simulink model "P702_NI_SoftECU"  (R2019a)
settings: Solver=ode1  StartTime=0.0  StopTime=Inf  FixedStep=0.001  RelTol=1e-3  EnableMultiTasking=on
PreLoadFcn:
  | run '.\VeriStand_BlockSet\NIVeriStandAddPaths.m'
undefined symbols (not defined in the file or in its folder): magnitude
libraries: simulink x83, simulink_extras x1
(part 6 of 76)

== system P702_NI_SoftECU/Input/ABS_ESC/DesiredTorqBrk_2_0x214 ==
  Bus_Sig : BusCreator  Inputs=7
  PrplWhlRear_Tq_RqMn : S-Function  Priority=1  FunctionName=NIVeriStandIO  Parameters=width dtype portnum stime stype btype  SFunctionDeploymentMode=off  EnableBusSupport=off  mask(NI VeriStand Inport){portnum=1, width=-1, stime=-1, dtype=auto, stype=auto, btype=1}
      mask prompts: portnum "Port number:"; width "Port dimensions (-1 for dynamically sized):"; stime "Sample time (-1 for inherited):"; dtype "Data type:"; stype "Signal type:"; btype "Block type:"
      mask help: Use this inport on any level of nested subsystems to allow NI VeriStand software to map signals to it.
      mask init:
      | NIVeriStandIO_init;
      settings: CopyFcn=NIVeriStand_MDL_functions('', 'IO_copy');  DeleteFcn=NIVeriStand_MDL_functions('', 'IO_delete');  MoveFcn=set_param(gcb, 'Mask', 'on');
      mask Callback portnum: NIVeriStand_MDL_functions('', 'IO_setportnum');
      mask TypeOptions dtype: auto | double | single | int8 | uint8 | int16 | uint16 | int32 | uint32 | boolean
      mask Callback dtype: NIVeriStand_MDL_functions('', 'IO_booleansignal');
      mask TypeOptions stype: auto | real | complex
      mask Display:
      | patch([-x x], [-y y], [.90980 .81960 .32156]);
      | plot([xrad -x x xrad], [yrad -y y yrad]);
      | fprintf('NI In%d', portnum);
  PrplWhlRear_Tq_RqMx : S-Function  Priority=2  FunctionName=NIVeriStandIO  Parameters=width dtype portnum stime stype btype  SFunctionDeploymentMode=off  EnableBusSupport=off  mask(NI VeriStand Inport){portnum=2, width=-1, stime=-1, dtype=auto, stype=auto, btype=1}
      mask prompts: portnum "Port number:"; width "Port dimensions (-1 for dynamically sized):"; stime "Sample time (-1 for inherited):"; dtype "Data type:"; stype "Signal type:"; btype "Block type:"
      mask help: Use this inport on any level of nested subsystems to allow NI VeriStand software to map signals to it.
      mask init:
      | NIVeriStandIO_init;
      settings: CopyFcn=NIVeriStand_MDL_functions('', 'IO_copy');  DeleteFcn=NIVeriStand_MDL_functions('', 'IO_delete');  MoveFcn=set_param(gcb, 'Mask', 'on');
      mask Callback portnum: NIVeriStand_MDL_functions('', 'IO_setportnum');
      mask TypeOptions dtype: auto | double | single | int8 | uint8 | int16 | uint16 | int32 | uint32 | boolean
      mask Callback dtype: NIVeriStand_MDL_functions('', 'IO_booleansignal');
      mask TypeOptions stype: auto | real | complex
      mask Display:
      | patch([-x x], [-y y], [.90980 .81960 .32156]);
      | plot([xrad -x x xrad], [yrad -y y yrad]);
      | fprintf('NI In%d', portnum);
  PrplWhlTot_Tq_RqMn : S-Function  Priority=3  FunctionName=NIVeriStandIO  Parameters=width dtype portnum stime stype btype  SFunctionDeploymentMode=off  EnableBusSupport=off  mask(NI VeriStand Inport){portnum=3, width=-1, stime=-1, dtype=auto, stype=auto, btype=1}
      mask prompts: portnum "Port number:"; width "Port dimensions (-1 for dynamically sized):"; stime "Sample time (-1 for inherited):"; dtype "Data type:"; stype "Signal type:"; btype "Block type:"
      mask help: Use this inport on any level of nested subsystems to allow NI VeriStand software to map signals to it.
      mask init:
      | NIVeriStandIO_init;
      settings: CopyFcn=NIVeriStand_MDL_functions('', 'IO_copy');  DeleteFcn=NIVeriStand_MDL_functions('', 'IO_delete');  MoveFcn=set_param(gcb, 'Mask', 'on');
      mask Callback portnum: NIVeriStand_MDL_functions('', 'IO_setportnum');
      mask TypeOptions dtype: auto | double | single | int8 | uint8 | int16 | uint16 | int32 | uint32 | boolean
      mask Callback dtype: NIVeriStand_MDL_functions('', 'IO_booleansignal');
      mask TypeOptions stype: auto | real | complex
      mask Display:
      | patch([-x x], [-y y], [.90980 .81960 .32156]);
      | plot([xrad -x x xrad], [yrad -y y yrad]);
      | fprintf('NI In%d', portnum);
  PrplWhlTqRqMn_No_Cnt : S-Function  Priority=4  FunctionName=NIVeriStandIO  Parameters=width dtype portnum stime stype btype  SFunctionDeploymentMode=off  EnableBusSupport=off  mask(NI VeriStand Inport){portnum=4, width=-1, stime=-1, dtype=auto, stype=auto, btype=1}
      mask prompts: portnum "Port number:"; width "Port dimensions (-1 for dynamically sized):"; stime "Sample time (-1 for inherited):"; dtype "Data type:"; stype "Signal type:"; btype "Block type:"
      mask help: Use this inport on any level of nested subsystems to allow NI VeriStand software to map signals to it.
      mask init:
      | NIVeriStandIO_init;
      settings: CopyFcn=NIVeriStand_MDL_functions('', 'IO_copy');  DeleteFcn=NIVeriStand_MDL_functions('', 'IO_delete');  MoveFcn=set_param(gcb, 'Mask', 'on');
      mask Callback portnum: NIVeriStand_MDL_functions('', 'IO_setportnum');
      mask TypeOptions dtype: auto | double | single | int8 | uint8 | int16 | uint16 | int32 | uint32 | boolean
      mask Callback dtype: NIVeriStand_MDL_functions('', 'IO_booleansignal');
      mask TypeOptions stype: auto | real | complex
      mask Display:
      | patch([-x x], [-y y], [.90980 .81960 .32156]);
      | plot([xrad -x x xrad], [yrad -y y yrad]);
      | fprintf('NI In%d', portnum);
  PrplWhlTqRqMn_No_Cs : S-Function  Priority=5  FunctionName=NIVeriStandIO  Parameters=width dtype portnum stime stype btype  SFunctionDeploymentMode=off  EnableBusSupport=off  mask(NI VeriStand Inport){portnum=5, width=-1, stime=-1, dtype=auto, stype=auto, btype=1}
      mask prompts: portnum "Port number:"; width "Port dimensions (-1 for dynamically sized):"; stime "Sample time (-1 for inherited):"; dtype "Data type:"; stype "Signal type:"; btype "Block type:"
      mask help: Use this inport on any level of nested subsystems to allow NI VeriStand software to map signals to it.
      mask init:
      | NIVeriStandIO_init;
      settings: CopyFcn=NIVeriStand_MDL_functions('', 'IO_copy');  DeleteFcn=NIVeriStand_MDL_functions('', 'IO_delete');  MoveFcn=set_param(gcb, 'Mask', 'on');
      mask Callback portnum: NIVeriStand_MDL_functions('', 'IO_setportnum');
      mask TypeOptions dtype: auto | double | single | int8 | uint8 | int16 | uint16 | int32 | uint32 | boolean
      mask Callback dtype: NIVeriStand_MDL_functions('', 'IO_booleansignal');
      mask TypeOptions stype: auto | real | complex
      mask Display:
      | patch([-x x], [-y y], [.90980 .81960 .32156]);
      | plot([xrad -x x xrad], [yrad -y y yrad]);
      | fprintf('NI In%d', portnum);
  RgenBrkDynoMde_B_Actl : S-Function  Priority=6  FunctionName=NIVeriStandIO  Parameters=width dtype portnum stime stype btype  SFunctionDeploymentMode=off  EnableBusSupport=off  mask(NI VeriStand Inport){portnum=6, width=-1, stime=-1, dtype=auto, stype=auto, btype=1}
      mask prompts: portnum "Port number:"; width "Port dimensions (-1 for dynamically sized):"; stime "Sample time (-1 for inherited):"; dtype "Data type:"; stype "Signal type:"; btype "Block type:"
      mask help: Use this inport on any level of nested subsystems to allow NI VeriStand software to map signals to it.
      mask init:
      | NIVeriStandIO_init;
      settings: CopyFcn=NIVeriStand_MDL_functions('', 'IO_copy');  DeleteFcn=NIVeriStand_MDL_functions('', 'IO_delete');  MoveFcn=set_param(gcb, 'Mask', 'on');
      mask Callback portnum: NIVeriStand_MDL_functions('', 'IO_setportnum');
      mask TypeOptions dtype: auto | double | single | int8 | uint8 | int16 | uint16 | int32 | uint32 | boolean
      mask Callback dtype: NIVeriStand_MDL_functions('', 'IO_booleansignal');
      mask TypeOptions stype: auto | real | complex
      mask Display:
      | patch([-x x], [-y y], [.90980 .81960 .32156]);
      | plot([xrad -x x xrad], [yrad -y y yrad]);
      | fprintf('NI In%d', portnum);
  RgenTqFalt_B_Actl : S-Function  Priority=7  FunctionName=NIVeriStandIO  Parameters=width dtype portnum stime stype btype  SFunctionDeploymentMode=off  EnableBusSupport=off  mask(NI VeriStand Inport){portnum=7, width=-1, stime=-1, dtype=auto, stype=auto, btype=1}
      mask prompts: portnum "Port number:"; width "Port dimensions (-1 for dynamically sized):"; stime "Sample time (-1 for inherited):"; dtype "Data type:"; stype "Signal type:"; btype "Block type:"
      mask help: Use this inport on any level of nested subsystems to allow NI VeriStand software to map signals to it.
      mask init:
      | NIVeriStandIO_init;
      settings: CopyFcn=NIVeriStand_MDL_functions('', 'IO_copy');  DeleteFcn=NIVeriStand_MDL_functions('', 'IO_delete');  MoveFcn=set_param(gcb, 'Mask', 'on');
      mask Callback portnum: NIVeriStand_MDL_functions('', 'IO_setportnum');
      mask TypeOptions dtype: auto | double | single | int8 | uint8 | int16 | uint16 | int32 | uint32 | boolean
      mask Callback dtype: NIVeriStand_MDL_functions('', 'IO_booleansignal');
      mask TypeOptions stype: auto | real | complex
      mask Display:
      | patch([-x x], [-y y], [.90980 .81960 .32156]);
      | plot([xrad -x x xrad], [yrad -y y yrad]);
      | fprintf('NI In%d', portnum);
  DesiredTorqBrk_2_0x214 : Outport
  wires:
  RgenBrkDynoMde_B_Actl/1 -> Bus_Sig/7  "RgenBrkDynoMde_B_Actl"
  RgenTqFalt_B_Actl/1 -> Bus_Sig/6  "RgenTqFalt_B_Actl"
  PrplWhlTqRqMn_No_Cnt/1 -> Bus_Sig/5  "PrplWhlTqRqMn_No_Cnt"
  PrplWhlTqRqMn_No_Cs/1 -> Bus_Sig/4  "PrplWhlTqRqMn_No_Cs"
  PrplWhlRear_Tq_RqMn/1 -> Bus_Sig/3  "PrplWhlRear_Tq_RqMn"
  PrplWhlRear_Tq_RqMx/1 -> Bus_Sig/2  "PrplWhlRear_Tq_RqMx"
  PrplWhlTot_Tq_RqMn/1 -> Bus_Sig/1  "PrplWhlTot_Tq_RqMn"
  Bus_Sig/1 -> DesiredTorqBrk_2_0x214/1  "DesiredTorqBrk_2_0x214"

== system P702_NI_SoftECU/Input/ABS_ESC/Global_PATS_SubTarget_0x49 ==
  Bus_Sig : BusCreator  Inputs=2
  immoSubTarget1Cmd_T1 : Constant  Commented=on  Value=0
  immoSubTarget1Data_T1 : Constant  Commented=on  Value=0
  Global_PATS_SubTarget_0x49 : Outport
  wires:
  immoSubTarget1Data_T1/1 -> Bus_Sig/2  "immoSubTarget1Data_T1"
  immoSubTarget1Cmd_T1/1 -> Bus_Sig/1  "immoSubTarget1Cmd_T1"
  Bus_Sig/1 -> Global_PATS_SubTarget_0x49/1  "Global_PATS_SubTarget_0x49"

== system P702_NI_SoftECU/Input/ABS_ESC/SelectDriveModeData2_0x44E ==
  Bus_Sig : BusCreator  Inputs=12
  SelDrvMdePos01_D_Stat : Constant  Commented=on  Value=31
  SelDrvMdePos02_D_Stat : Constant  Commented=on  Value=31
  SelDrvMdePos03_D_Stat : Constant  Commented=on  Value=31
  SelDrvMdePos04_D_Stat : Constant  Commented=on  Value=31
  SelDrvMdePos05_D_Stat : Constant  Commented=on  Value=31
  SelDrvMdePos06_D_Stat : Constant  Commented=on  Value=31
  SelDrvMdePos07_D_Stat : Constant  Commented=on  Value=31
  SelDrvMdePos08_D_Stat : Constant  Commented=on  Value=31
  SelDrvMdePos09_D_Stat : Constant  Commented=on  Value=31
  SelDrvMdePos10_D_Stat : Constant  Commented=on  Value=31
  SelDrvMdePos11_D_Stat : Constant  Commented=on  Value=31
  SelDrvMdePos12_D_Stat : Constant  Commented=on  Value=31
  SelectDriveModeData2_0x44E : Outport
  wires:
  SelDrvMdePos08_D_Stat/1 -> Bus_Sig/12  "SelDrvMdePos08_D_Stat"
  SelDrvMdePos09_D_Stat/1 -> Bus_Sig/11  "SelDrvMdePos09_D_Stat"
  SelDrvMdePos10_D_Stat/1 -> Bus_Sig/10  "SelDrvMdePos10_D_Stat"
  SelDrvMdePos11_D_Stat/1 -> Bus_Sig/9  "SelDrvMdePos11_D_Stat"
  SelDrvMdePos12_D_Stat/1 -> Bus_Sig/8  "SelDrvMdePos12_D_Stat"
  SelDrvMdePos07_D_Stat/1 -> Bus_Sig/7  "SelDrvMdePos07_D_Stat"
  SelDrvMdePos06_D_Stat/1 -> Bus_Sig/6  "SelDrvMdePos06_D_Stat"
  SelDrvMdePos05_D_Stat/1 -> Bus_Sig/5  "SelDrvMdePos05_D_Stat"
  SelDrvMdePos04_D_Stat/1 -> Bus_Sig/4  "SelDrvMdePos04_D_Stat"
  SelDrvMdePos03_D_Stat/1 -> Bus_Sig/3  "SelDrvMdePos03_D_Stat"
  SelDrvMdePos02_D_Stat/1 -> Bus_Sig/2  "SelDrvMdePos02_D_Stat"
  SelDrvMdePos01_D_Stat/1 -> Bus_Sig/1  "SelDrvMdePos01_D_Stat"
  Bus_Sig/1 -> SelectDriveModeData2_0x44E/1  "SelectDriveModeData2_0x44E"

== system P702_NI_SoftECU/Input/ABS_ESC/SelectDriveModeData_0x420 ==
  ActvDrvMde_D2_Stat : Constant  Commented=on  Value=31
  AwdMde_D_RqBrk : Constant  Commented=on  Value=5
  Bus_Sig : BusCreator  Inputs=18
  SelDrvMdeMsgTxt_D_Rq : Constant  Commented=on  Value=0
  SelDrvMdePos01_B_Avail : Constant  Commented=on  Value=0
  SelDrvMdePos02_B_Avail : Constant  Commented=on  Value=0
  SelDrvMdePos03_B_Avail : Constant  Commented=on  Value=0
  SelDrvMdePos04_B_Avail : Constant  Commented=on  Value=0
  SelDrvMdePos05_B_Avail : Constant  Commented=on  Value=0
  SelDrvMdePos06_B_Avail : Constant  Commented=on  Value=0
  SelDrvMdePos07_B_Avail : Constant  Commented=on  Value=0
  SelDrvMdePos08_B_Avail : Constant  Commented=on  Value=0
  SelDrvMdePos09_B_Avail : Constant  Commented=on  Value=0
  SelDrvMdePos10_B_Avail : Constant  Commented=on  Value=0
  SelDrvMdePos11_B_Avail : Constant  Commented=on  Value=0
  SelDrvMdePos12_B_Avail : Constant  Commented=on  Value=0
  SelDrvMdePt_D_Rq : Constant  Commented=on  Value=0
  SelDrvMde_D2_Rq : Constant  Commented=on  Value=31
  SelDrvMde_D_Stat : Constant  Commented=on  Value=0
  SelectDriveModeData_0x420 : Outport
  wires:
  SelDrvMde_D2_Rq/1 -> Bus_Sig/18  "SelDrvMde_D2_Rq"
  ActvDrvMde_D2_Stat/1 -> Bus_Sig/17  "ActvDrvMde_D2_Stat"
  SelDrvMdePos12_B_Avail/1 -> Bus_Sig/16  "SelDrvMdePos12_B_Avail"
  SelDrvMdePos11_B_Avail/1 -> Bus_Sig/15  "SelDrvMdePos11_B_Avail"
  SelDrvMdePos10_B_Avail/1 -> Bus_Sig/14  "SelDrvMdePos10_B_Avail"
  SelDrvMdePos09_B_Avail/1 -> Bus_Sig/13  "SelDrvMdePos09_B_Avail"
  SelDrvMdePos08_B_Avail/1 -> Bus_Sig/12  "SelDrvMdePos08_B_Avail"
  SelDrvMdePos07_B_Avail/1 -> Bus_Sig/11  "SelDrvMdePos07_B_Avail"
  SelDrvMdePos06_B_Avail/1 -> Bus_Sig/10  "SelDrvMdePos06_B_Avail"
  SelDrvMdePos05_B_Avail/1 -> Bus_Sig/9  "SelDrvMdePos05_B_Avail"
  SelDrvMdePos04_B_Avail/1 -> Bus_Sig/8  "SelDrvMdePos04_B_Avail"
  SelDrvMdePos03_B_Avail/1 -> Bus_Sig/7  "SelDrvMdePos03_B_Avail"
  SelDrvMdePos02_B_Avail/1 -> Bus_Sig/6  "SelDrvMdePos02_B_Avail"
  AwdMde_D_RqBrk/1 -> Bus_Sig/5  "AwdMde_D_RqBrk"
  SelDrvMdePos01_B_Avail/1 -> Bus_Sig/4  "SelDrvMdePos01_B_Avail"
  SelDrvMde_D_Stat/1 -> Bus_Sig/3  "SelDrvMde_D_Stat"
  SelDrvMdePt_D_Rq/1 -> Bus_Sig/2  "SelDrvMdePt_D_Rq"
  SelDrvMdeMsgTxt_D_Rq/1 -> Bus_Sig/1  "SelDrvMdeMsgTxt_D_Rq"
  Bus_Sig/1 -> SelectDriveModeData_0x420/1  "SelectDriveModeData_0x420"

== system P702_NI_SoftECU/Input/ABS_ESC/SteeringPinion_Data2_0x7F ==
  AwdLatDelta_B_Rq_In : S-Function  Priority=1  FunctionName=NIVeriStandIO  Parameters=width dtype portnum stime stype btype  SFunctionDeploymentMode=off  EnableBusSupport=off  mask(NI VeriStand Inport){portnum=1, width=-1, stime=-1, dtype=auto, stype=auto, btype=1}
      mask prompts: portnum "Port number:"; width "Port dimensions (-1 for dynamically sized):"; stime "Sample time (-1 for inherited):"; dtype "Data type:"; stype "Signal type:"; btype "Block type:"
      mask help: Use this inport on any level of nested subsystems to allow NI VeriStand software to map signals to it.
      mask init:
      | NIVeriStandIO_init;
      settings: CopyFcn=NIVeriStand_MDL_functions('', 'IO_copy');  DeleteFcn=NIVeriStand_MDL_functions('', 'IO_delete');  MoveFcn=set_param(gcb, 'Mask', 'on');
      mask Callback portnum: NIVeriStand_MDL_functions('', 'IO_setportnum');
      mask TypeOptions dtype: auto | double | single | int8 | uint8 | int16 | uint16 | int32 | uint32 | boolean
      mask Callback dtype: NIVeriStand_MDL_functions('', 'IO_booleansignal');
      mask TypeOptions stype: auto | real | complex
      mask Display:
      | patch([-x x], [-y y], [.90980 .81960 .32156]);
      | plot([xrad -x x xrad], [yrad -y y yrad]);
      | fprintf('NI In%d', portnum);
  AwdLatDelta_Tq_Rq_In : S-Function  Priority=2  FunctionName=NIVeriStandIO  Parameters=width dtype portnum stime stype btype  SFunctionDeploymentMode=off  EnableBusSupport=off  mask(NI VeriStand Inport){portnum=2, width=-1, stime=-1, dtype=auto, stype=auto, btype=1}
      mask prompts: portnum "Port number:"; width "Port dimensions (-1 for dynamically sized):"; stime "Sample time (-1 for inherited):"; dtype "Data type:"; stype "Signal type:"; btype "Block type:"
      mask help: Use this inport on any level of nested subsystems to allow NI VeriStand software to map signals to it.
      mask init:
      | NIVeriStandIO_init;
      settings: CopyFcn=NIVeriStand_MDL_functions('', 'IO_copy');  DeleteFcn=NIVeriStand_MDL_functions('', 'IO_delete');  MoveFcn=set_param(gcb, 'Mask', 'on');
      mask Callback portnum: NIVeriStand_MDL_functions('', 'IO_setportnum');
      mask TypeOptions dtype: auto | double | single | int8 | uint8 | int16 | uint16 | int32 | uint32 | boolean
      mask Callback dtype: NIVeriStand_MDL_functions('', 'IO_booleansignal');
      mask TypeOptions stype: auto | real | complex
      mask Display:
      | patch([-x x], [-y y], [.90980 .81960 .32156]);
      | plot([xrad -x x xrad], [yrad -y y yrad]);
      | fprintf('NI In%d', portnum);
  Bus_Sig : BusCreator  Inputs=2
  SteeringPinion_Data2_0x7F : Outport
  wires:
  AwdLatDelta_Tq_Rq_In/1 -> Bus_Sig/2  "AwdLatDelta_Tq_Rq"
  AwdLatDelta_B_Rq_In/1 -> Bus_Sig/1  "AwdLatDelta_B_Rq"
  Bus_Sig/1 -> SteeringPinion_Data2_0x7F/1  "SteeringPinion_Data2_0x7F"

== system P702_NI_SoftECU/Input/ABS_ESC/TesterPhysicalResABS_0x768 ==
  Bus_Sig : BusCreator  Inputs=1
  TesterPhysicalResABS : Constant  Commented=on  Value=0
  TesterPhysicalResABS_0x768 : Outport
  wires:
  TesterPhysicalResABS/1 -> Bus_Sig/1  "TesterPhysicalResABS"
  Bus_Sig/1 -> TesterPhysicalResABS_0x768/1  "TesterPhysicalResABS_0x768"

== system P702_NI_SoftECU/Input/ABS_ESC/TrailerBrakeData_0x412 ==
  Bus_Sig : BusCreator  Inputs=3
  TrlrBrk_Pc_Rq : Constant  Commented=on  Value=0
  VehPtch_An_Dsply : Constant  Commented=on  Value=-64
  VehRol_An_Dsply : Constant  Commented=on  Value=-64
  TrailerBrakeData_0x412 : Outport
  wires:
  Bus_Sig/1 -> TrailerBrakeData_0x412/1  "TrailerBrakeData_0x412"
  TrlrBrk_Pc_Rq/1 -> Bus_Sig/1  "TrlrBrk_Pc_Rq"
  VehPtch_An_Dsply/1 -> Bus_Sig/2  "VehPtch_An_Dsply"
  VehRol_An_Dsply/1 -> Bus_Sig/3  "VehRol_An_Dsply"

== system P702_NI_SoftECU/Input/ABS_ESC/WheelData_0x216 ==
  BrkObdData_No_Actl : S-Function  Priority=1  FunctionName=NIVeriStandIO  Parameters=width dtype portnum stime stype btype  SFunctionDeploymentMode=off  EnableBusSupport=off  mask(NI VeriStand Inport){portnum=1, width=-1, stime=-1, dtype=auto, stype=auto, btype=1}
      mask prompts: portnum "Port number:"; width "Port dimensions (-1 for dynamically sized):"; stime "Sample time (-1 for inherited):"; dtype "Data type:"; stype "Signal type:"; btype "Block type:"
      mask help: Use this inport on any level of nested subsystems to allow NI VeriStand software to map signals to it.
      mask init:
      | NIVeriStandIO_init;
      settings: CopyFcn=NIVeriStand_MDL_functions('', 'IO_copy');  DeleteFcn=NIVeriStand_MDL_functions('', 'IO_delete');  MoveFcn=set_param(gcb, 'Mask', 'on');
      mask Callback portnum: NIVeriStand_MDL_functions('', 'IO_setportnum');
      mask TypeOptions dtype: auto | double | single | int8 | uint8 | int16 | uint16 | int32 | uint32 | boolean
      mask Callback dtype: NIVeriStand_MDL_functions('', 'IO_booleansignal');
      mask TypeOptions stype: auto | real | complex
      mask Display:
      | patch([-x x], [-y y], [.90980 .81960 .32156]);
      | plot([xrad -x x xrad], [yrad -y y yrad]);
      | fprintf('NI In%d', portnum);
  BrkObdIndex_No_Actl : S-Function  Priority=2  FunctionName=NIVeriStandIO  Parameters=width dtype portnum stime stype btype  SFunctionDeploymentMode=off  EnableBusSupport=off  mask(NI VeriStand Inport){portnum=2, width=-1, stime=-1, dtype=auto, stype=auto, btype=1}
      mask prompts: portnum "Port number:"; width "Port dimensions (-1 for dynamically sized):"; stime "Sample time (-1 for inherited):"; dtype "Data type:"; stype "Signal type:"; btype "Block type:"
      mask help: Use this inport on any level of nested subsystems to allow NI VeriStand software to map signals to it.
      mask init:
      | NIVeriStandIO_init;
      settings: CopyFcn=NIVeriStand_MDL_functions('', 'IO_copy');  DeleteFcn=NIVeriStand_MDL_functions('', 'IO_delete');  MoveFcn=set_param(gcb, 'Mask', 'on');
      mask Callback portnum: NIVeriStand_MDL_functions('', 'IO_setportnum');
      mask TypeOptions dtype: auto | double | single | int8 | uint8 | int16 | uint16 | int32 | uint32 | boolean
      mask Callback dtype: NIVeriStand_MDL_functions('', 'IO_booleansignal');
      mask TypeOptions stype: auto | real | complex
      mask Display:
      | patch([-x x], [-y y], [.90980 .81960 .32156]);
      | plot([xrad -x x xrad], [yrad -y y yrad]);
      | fprintf('NI In%d', portnum);
  Bus_Sig : BusCreator  Inputs=10
  WhlDirFl_D_Actl_In : S-Function  Priority=3  FunctionName=NIVeriStandIO  Parameters=width dtype portnum stime stype btype  SFunctionDeploymentMode=off  EnableBusSupport=off  mask(NI VeriStand Inport){portnum=3, width=-1, stime=-1, dtype=auto, stype=auto, btype=1}
      mask prompts: portnum "Port number:"; width "Port dimensions (-1 for dynamically sized):"; stime "Sample time (-1 for inherited):"; dtype "Data type:"; stype "Signal type:"; btype "Block type:"
      mask help: Use this inport on any level of nested subsystems to allow NI VeriStand software to map signals to it.
      mask init:
      | NIVeriStandIO_init;
      settings: CopyFcn=NIVeriStand_MDL_functions('', 'IO_copy');  DeleteFcn=NIVeriStand_MDL_functions('', 'IO_delete');  MoveFcn=set_param(gcb, 'Mask', 'on');
      mask Callback portnum: NIVeriStand_MDL_functions('', 'IO_setportnum');
      mask TypeOptions dtype: auto | double | single | int8 | uint8 | int16 | uint16 | int32 | uint32 | boolean
      mask Callback dtype: NIVeriStand_MDL_functions('', 'IO_booleansignal');
      mask TypeOptions stype: auto | real | complex
      mask Display:
      | patch([-x x], [-y y], [.90980 .81960 .32156]);
      | plot([xrad -x x xrad], [yrad -y y yrad]);
      | fprintf('NI In%d', portnum);
  WhlDirFr_D_Actl_In : S-Function  Priority=4  FunctionName=NIVeriStandIO  Parameters=width dtype portnum stime stype btype  SFunctionDeploymentMode=off  EnableBusSupport=off  mask(NI VeriStand Inport){portnum=4, width=-1, stime=-1, dtype=auto, stype=auto, btype=1}
      mask prompts: portnum "Port number:"; width "Port dimensions (-1 for dynamically sized):"; stime "Sample time (-1 for inherited):"; dtype "Data type:"; stype "Signal type:"; btype "Block type:"
      mask help: Use this inport on any level of nested subsystems to allow NI VeriStand software to map signals to it.
      mask init:
      | NIVeriStandIO_init;
      settings: CopyFcn=NIVeriStand_MDL_functions('', 'IO_copy');  DeleteFcn=NIVeriStand_MDL_functions('', 'IO_delete');  MoveFcn=set_param(gcb, 'Mask', 'on');
      mask Callback portnum: NIVeriStand_MDL_functions('', 'IO_setportnum');
      mask TypeOptions dtype: auto | double | single | int8 | uint8 | int16 | uint16 | int32 | uint32 | boolean
      mask Callback dtype: NIVeriStand_MDL_functions('', 'IO_booleansignal');
      mask TypeOptions stype: auto | real | complex
      mask Display:
      | patch([-x x], [-y y], [.90980 .81960 .32156]);
      | plot([xrad -x x xrad], [yrad -y y yrad]);
      | fprintf('NI In%d', portnum);
  WhlDirRl_D_Actl : S-Function  Priority=5  FunctionName=NIVeriStandIO  Parameters=width dtype portnum stime stype btype  SFunctionDeploymentMode=off  EnableBusSupport=off  mask(NI VeriStand Inport){portnum=5, width=-1, stime=-1, dtype=auto, stype=auto, btype=1}
      mask prompts: portnum "Port number:"; width "Port dimensions (-1 for dynamically sized):"; stime "Sample time (-1 for inherited):"; dtype "Data type:"; stype "Signal type:"; btype "Block type:"
      mask help: Use this inport on any level of nested subsystems to allow NI VeriStand software to map signals to it.
      mask init:
      | NIVeriStandIO_init;
      settings: CopyFcn=NIVeriStand_MDL_functions('', 'IO_copy');  DeleteFcn=NIVeriStand_MDL_functions('', 'IO_delete');  MoveFcn=set_param(gcb, 'Mask', 'on');
      mask Callback portnum: NIVeriStand_MDL_functions('', 'IO_setportnum');
      mask TypeOptions dtype: auto | double | single | int8 | uint8 | int16 | uint16 | int32 | uint32 | boolean
      mask Callback dtype: NIVeriStand_MDL_functions('', 'IO_booleansignal');
      mask TypeOptions stype: auto | real | complex
      mask Display:
      | patch([-x x], [-y y], [.90980 .81960 .32156]);
      | plot([xrad -x x xrad], [yrad -y y yrad]);
      | fprintf('NI In%d', portnum);
  WhlDirRr_D_Actl : S-Function  Priority=6  FunctionName=NIVeriStandIO  Parameters=width dtype portnum stime stype btype  SFunctionDeploymentMode=off  EnableBusSupport=off  mask(NI VeriStand Inport){portnum=6, width=-1, stime=-1, dtype=auto, stype=auto, btype=1}
      mask prompts: portnum "Port number:"; width "Port dimensions (-1 for dynamically sized):"; stime "Sample time (-1 for inherited):"; dtype "Data type:"; stype "Signal type:"; btype "Block type:"
      mask help: Use this inport on any level of nested subsystems to allow NI VeriStand software to map signals to it.
      mask init:
      | NIVeriStandIO_init;
      settings: CopyFcn=NIVeriStand_MDL_functions('', 'IO_copy');  DeleteFcn=NIVeriStand_MDL_functions('', 'IO_delete');  MoveFcn=set_param(gcb, 'Mask', 'on');
      mask Callback portnum: NIVeriStand_MDL_functions('', 'IO_setportnum');
      mask TypeOptions dtype: auto | double | single | int8 | uint8 | int16 | uint16 | int32 | uint32 | boolean
      mask Callback dtype: NIVeriStand_MDL_functions('', 'IO_booleansignal');
      mask TypeOptions stype: auto | real | complex
      mask Display:
      | patch([-x x], [-y y], [.90980 .81960 .32156]);
      | plot([xrad -x x xrad], [yrad -y y yrad]);
      | fprintf('NI In%d', portnum);
  WhlRotatFl_No_Cnt_In : S-Function  Priority=7  FunctionName=NIVeriStandIO  Parameters=width dtype portnum stime stype btype  SFunctionDeploymentMode=off  EnableBusSupport=off  mask(NI VeriStand Inport){portnum=7, width=-1, stime=-1, dtype=auto, stype=auto, btype=1}
      mask prompts: portnum "Port number:"; width "Port dimensions (-1 for dynamically sized):"; stime "Sample time (-1 for inherited):"; dtype "Data type:"; stype "Signal type:"; btype "Block type:"
      mask help: Use this inport on any level of nested subsystems to allow NI VeriStand software to map signals to it.
      mask init:
      | NIVeriStandIO_init;
      settings: CopyFcn=NIVeriStand_MDL_functions('', 'IO_copy');  DeleteFcn=NIVeriStand_MDL_functions('', 'IO_delete');  MoveFcn=set_param(gcb, 'Mask', 'on');
      mask Callback portnum: NIVeriStand_MDL_functions('', 'IO_setportnum');
      mask TypeOptions dtype: auto | double | single | int8 | uint8 | int16 | uint16 | int32 | uint32 | boolean
      mask Callback dtype: NIVeriStand_MDL_functions('', 'IO_booleansignal');
      mask TypeOptions stype: auto | real | complex
      mask Display:
      | patch([-x x], [-y y], [.90980 .81960 .32156]);
      | plot([xrad -x x xrad], [yrad -y y yrad]);
      | fprintf('NI In%d', portnum);
  WhlRotatFr_No_Cnt_In : S-Function  Priority=8  FunctionName=NIVeriStandIO  Parameters=width dtype portnum stime stype btype  SFunctionDeploymentMode=off  EnableBusSupport=off  mask(NI VeriStand Inport){portnum=8, width=-1, stime=-1, dtype=auto, stype=auto, btype=1}
      mask prompts: portnum "Port number:"; width "Port dimensions (-1 for dynamically sized):"; stime "Sample time (-1 for inherited):"; dtype "Data type:"; stype "Signal type:"; btype "Block type:"
      mask help: Use this inport on any level of nested subsystems to allow NI VeriStand software to map signals to it.
      mask init:
      | NIVeriStandIO_init;
      settings: CopyFcn=NIVeriStand_MDL_functions('', 'IO_copy');  DeleteFcn=NIVeriStand_MDL_functions('', 'IO_delete');  MoveFcn=set_param(gcb, 'Mask', 'on');
      mask Callback portnum: NIVeriStand_MDL_functions('', 'IO_setportnum');
      mask TypeOptions dtype: auto | double | single | int8 | uint8 | int16 | uint16 | int32 | uint32 | boolean
      mask Callback dtype: NIVeriStand_MDL_functions('', 'IO_booleansignal');
      mask TypeOptions stype: auto | real | complex
      mask Display:
      | patch([-x x], [-y y], [.90980 .81960 .32156]);
      | plot([xrad -x x xrad], [yrad -y y yrad]);
      | fprintf('NI In%d', portnum);
  WhlRotatRl_No_Cnt_In : S-Function  Priority=9  FunctionName=NIVeriStandIO  Parameters=width dtype portnum stime stype btype  SFunctionDeploymentMode=off  EnableBusSupport=off  mask(NI VeriStand Inport){portnum=9, width=-1, stime=-1, dtype=auto, stype=auto, btype=1}
      mask prompts: portnum "Port number:"; width "Port dimensions (-1 for dynamically sized):"; stime "Sample time (-1 for inherited):"; dtype "Data type:"; stype "Signal type:"; btype "Block type:"
      mask help: Use this inport on any level of nested subsystems to allow NI VeriStand software to map signals to it.
      mask init:
      | NIVeriStandIO_init;
      settings: CopyFcn=NIVeriStand_MDL_functions('', 'IO_copy');  DeleteFcn=NIVeriStand_MDL_functions('', 'IO_delete');  MoveFcn=set_param(gcb, 'Mask', 'on');
      mask Callback portnum: NIVeriStand_MDL_functions('', 'IO_setportnum');
      mask TypeOptions dtype: auto | double | single | int8 | uint8 | int16 | uint16 | int32 | uint32 | boolean
      mask Callback dtype: NIVeriStand_MDL_functions('', 'IO_booleansignal');
      mask TypeOptions stype: auto | real | complex
      mask Display:
      | patch([-x x], [-y y], [.90980 .81960 .32156]);
      | plot([xrad -x x xrad], [yrad -y y yrad]);
      | fprintf('NI In%d', portnum);
  WhlRotatRr_No_Cnt_In : S-Function  Priority=10  FunctionName=NIVeriStandIO  Parameters=width dtype portnum stime stype btype  SFunctionDeploymentMode=off  EnableBusSupport=off  mask(NI VeriStand Inport){portnum=10, width=-1, stime=-1, dtype=auto, stype=auto, btype=1}
      mask prompts: portnum "Port number:"; width "Port dimensions (-1 for dynamically sized):"; stime "Sample time (-1 for inherited):"; dtype "Data type:"; stype "Signal type:"; btype "Block type:"
      mask help: Use this inport on any level of nested subsystems to allow NI VeriStand software to map signals to it.
      mask init:
      | NIVeriStandIO_init;
      settings: CopyFcn=NIVeriStand_MDL_functions('', 'IO_copy');  DeleteFcn=NIVeriStand_MDL_functions('', 'IO_delete');  MoveFcn=set_param(gcb, 'Mask', 'on');
      mask Callback portnum: NIVeriStand_MDL_functions('', 'IO_setportnum');
      mask TypeOptions dtype: auto | double | single | int8 | uint8 | int16 | uint16 | int32 | uint32 | boolean
      mask Callback dtype: NIVeriStand_MDL_functions('', 'IO_booleansignal');
      mask TypeOptions stype: auto | real | complex
      mask Display:
      | patch([-x x], [-y y], [.90980 .81960 .32156]);
      | plot([xrad -x x xrad], [yrad -y y yrad]);
      | fprintf('NI In%d', portnum);
  WheelData_0x216 : Outport
  wires:
  BrkObdData_No_Actl/1 -> Bus_Sig/10  "BrkObdData_No_Actl"
  BrkObdIndex_No_Actl/1 -> Bus_Sig/9  "BrkObdIndex_No_Actl"
  WhlDirRr_D_Actl/1 -> Bus_Sig/8  "WhlDirRr_D_Actl"
  WhlDirFl_D_Actl_In/1 -> Bus_Sig/7  "WhlDirFl_D_Actl"
  WhlDirFr_D_Actl_In/1 -> Bus_Sig/6  "WhlDirFr_D_Actl"
  WhlDirRl_D_Actl/1 -> Bus_Sig/5  "WhlDirRl_D_Actl"
  WhlRotatRl_No_Cnt_In/1 -> Bus_Sig/4  "WhlRotatRl_No_Cnt"
  WhlRotatRr_No_Cnt_In/1 -> Bus_Sig/3  "WhlRotatRr_No_Cnt"
  WhlRotatFl_No_Cnt_In/1 -> Bus_Sig/2  "WhlRotatFl_No_Cnt"
  WhlRotatFr_No_Cnt_In/1 -> Bus_Sig/1  "WhlRotatFr_No_Cnt"
  Bus_Sig/1 -> WheelData_0x216/1  "WheelData_0x216"

== system P702_NI_SoftECU/Input/ABS_ESC/WheelSpeed_0x217 ==
  Bus_Sig : BusCreator  Inputs=4
  Constant{1..4} (4 alike) : Constant  Value=0
  WheelSpeed_0x217 : Outport
  wires:
  Constant4/1 -> Bus_Sig/4  "WhlRr_W_Meas"
  Constant3/1 -> Bus_Sig/3  "WhlRl_W_Meas"
  Constant2/1 -> Bus_Sig/2  "WhlFr_W_Meas"
  Constant1/1 -> Bus_Sig/1  "WhlFl_W_Meas"
  Bus_Sig/1 -> WheelSpeed_0x217/1  "WheelSpeed_0x217"
